simulink model "BLDC_Motor"  (R2024a)
settings: Solver=VariableStepAuto  StartTime=0.0  StopTime=10.0  RelTol=1e-3
undefined symbols (not defined in the file): Ion, Lithium
libraries: spsMosfetLib x6, spsBatteryLib x1, slpidlib x1, spsPermanentMagnetSynchronousMachineLib x1, sps_lib x1
settings Model: SimulationMode=accelerator  Creator=RGUKT  LastModifiedBy=RGUKT

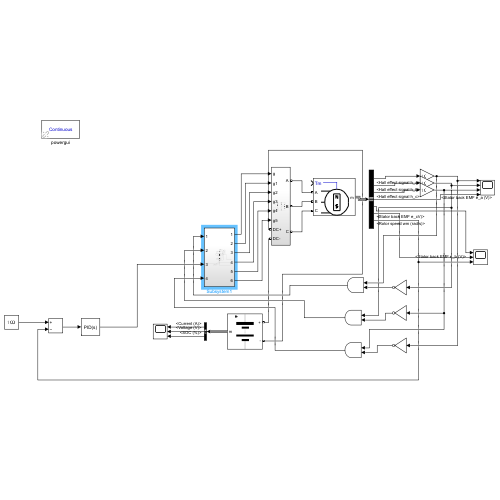
[thumbnail: Simulink's stored preview of the top-level diagram]
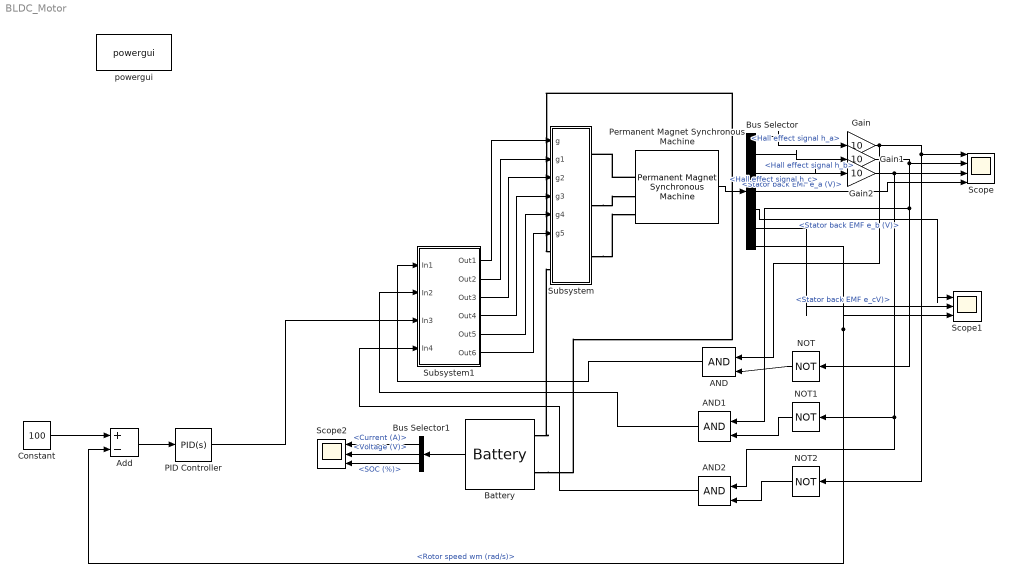
== system BLDC_Motor ==
  AND : Logic  IconShape=distinctive  AllPortsSameDT=off  OutDataTypeStr=boolean
  AND1 : Logic  IconShape=distinctive  AllPortsSameDT=off  OutDataTypeStr=boolean
  AND2 : Logic  IconShape=distinctive  AllPortsSameDT=off  OutDataTypeStr=boolean
  Add : Sum  Inputs=+-
  Battery : spsBatteryLib/Battery  BatType=Lithium-Ion  ShowTempParam=off  ThermalPreset=no  ShowAgeParam=off  NomV=7.2  NomQ=5.4  SOC=100  Batt_Tr=30  PresetModel=on  MaxQ=5.4  MinV=5.4  FullV=8.3807  Dis_rate=2.3478  R=0.013333  Normal_OP=4.8835  expZone="[7.7788      0.2653]"  current=[6.5 13 32.5]  Units=Time  Tci=20  NomT=20  T2=-30  MaxQ2=4.8  FullV2=7.1  Normal_OP2=5.655  expZone2="[6.58           1]"  Rca=0.6  ti=2000  Dp=0  Neq0=0  Tsim=1e6  Ta1=25  Qeol=5.4*0.9  Reol=0.013333*1.2  Char_age=[2.3478, 3]  Dis_age=[2.3478, 10]  N1=1500  N2=10500  N3=1000  N4=1400  Ta2=45  N5=950
  Bus Selector : BusSelector  OutputSignals=Hall effect signal h_a,Hall effect signal h_b,Hall effect signal h_c,Stator back EMF e_a (V),Stator back EMF e_b (V),Stator back EMF e_cV),Rotor speed wm (rad/s)
  Bus Selector1 : BusSelector  OutputSignals=Current (A),Voltage (V),SOC (%)
  Constant : Constant  Value=100
  Gain : Gain  Gain=10
  Gain1 : Gain  Gain=10
  Gain2 : Gain  Gain=10
  NOT : Logic  Operator=NOT  IconShape=distinctive  AllPortsSameDT=off  OutDataTypeStr=boolean
  NOT1 : Logic  Operator=NOT  IconShape=distinctive  AllPortsSameDT=off  OutDataTypeStr=boolean
  NOT2 : Logic  Operator=NOT  IconShape=distinctive  AllPortsSameDT=off  OutDataTypeStr=boolean
  PID Controller : slpidlib/PID Controller  Controller=PID  Form=Parallel  TimeDomain=Continuous-time  UseExternalTs=off  SampleTime=-1  IntegratorMethod=Forward Euler  FilterMethod=Forward Euler  ControllerParametersSource=internal  P=1  I=1  UseKiTs=off  D=0  UseExternalDerivativeSource=off  N=100  UseFilter=on  TunerSelectOption=Transfer Function Based (PID Tuner App)  InitialConditionSource=internal  InitialConditionForIntegrator=0  InitialConditionForFilter=0  DifferentiatorICPrevScaledInput=0  ExternalReset=none  TrackingMode=off  Kt=1  LimitOutput=off  SatLimitsSource=internal  UpperSaturationLimit=inf  LowerSaturationLimit=-inf  LinearizeAsGain=on  AntiWindupMode=none  Kb=1  LimitIntegrator=off  UpperIntegratorSaturationLimit=inf  LowerIntegratorSaturationLimit=-inf  POutMin=[]  POutMax=[]  IOutMin=[]  IOutMax=[]  DOutMin=[]  DOutMax=[]  NOutMin=[]  NOutMax=[]  SumOutMin=[]  SumOutMax=[]  SaturationOutMin=[]  SaturationOutMax=[]  PParamMin=[]  PParamMax=[]  IParamMin=[]  IParamMax=[]  DParamMin=[]  DParamMax=[]  NParamMin=[]  NParamMax=[]  KbParamMin=[]  KbParamMax=[]  KtParamMin=[]  KtParamMax=[]  KbOutMin=[]  KbOutMax=[]  KtOutMin=[]  KtOutMax=[]  IntegratorOutMin=[]  IntegratorOutMax=[]  FilterOutMin=[]  FilterOutMax=[]  SumI1OutMin=[]  SumI1OutMax=[]  SumI2OutMin=[]  SumI2OutMax=[]  SumI3OutMin=[]  SumI3OutMax=[]  SumI4OutMin=[]  SumI4OutMax=[]  SumDOutMin=[]  SumDOutMax=[]  DifferentiatorOutMin=[]  DifferentiatorOutMax=[]  FilterDiffOutCoefMin=[]  FilterDiffOutCoefMax=[]  ReciprocalOutMin=[]  ReciprocalOutMax=[]  SumDenOutMin=[]  SumDenOutMax=[]  SumNumOutMin=[]  SumNumOutMax=[]  DivideOutMin=[]  DivideOutMax=[]  UdiffTsProdOutMin=[]  UdiffTsProdOutMax=[]  NTsProdOutMin=[]  NTsProdOutMax=[]  UintegralTsProdOutMin=[]  UintegralTsProdOutMax=[]  UngainTsProdOutMin=[]  UngainTsProdOutMax=[]  ClampingZeroOutDataTypeStr=Inherit: Inherit via back propagation  ClampingZeroOutMin=[]  ClampingZeroOutMax=[]  FilterDenConstantOutDataTypeStr=Inherit: Inherit via back propagation  FilterDenConstantOutMin=[]  FilterDenConstantOutMax=[]  PCopyOutDataTypeStr=Inherit: Inherit via back propagation  PCopyOutMin=[]  PCopyOutMax=[]  NCopyOutDataTypeStr=Inherit: Inherit via back propagation  NCopyOutMin=[]  NCopyOutMax=[]  IntegratorContinuousStateAttributes=''  IntegratorStateMustResolveToSignalObject=off  IntegratorRTWStateStorageClass=Auto  FilterContinuousStateAttributes=''  FilterStateMustResolveToSignalObject=off  FilterRTWStateStorageClass=Auto  ParallelPVariant=InternalParameters  IdealPVariant=Disabled  IVariant=InternalParameters  DVariant=InternalParameters  IntegratorVariant=Continuous  SatVariant=Disabled  AWVariant=Passthrough  PCopyVariant=Disabled  TRVariant=Disabled  FdbkBlocksVariant=Forward  IdealPFdbkVariant=Disabled  SatFdbkVariant=Disabled  DerivativeFilterVariant=ContFilter  NVariant=InternalParameters  NCopyVariant=Disabled  FilterICVariant=InternalICsFilter  IntegratorICVariant=InternalICs  ExternalResetVariant=Disabled  TRSumVariant=Passthrough  SumFdbkVariant=Disabled  SumVariant=Sum_PID  TsampFilterVariant=InternalTs  TsampNgainVariant=Passthrough  TsampIntegralVariant=Disabled_SignalSpec  ExternalSaturationOutDataTypeStr=Inherit: Same as second input  DerivativeSourceVariant=ErrorSignal
  Permanent Magnet Synchronous Machine : spsPermanentMagnetSynchronousMachineLib/Permanent Magnet Synchronous Machine  NbPhases=3  FluxDistribution=Trapezoidal  RotorType=Round  MechanicalLoad=Torque Tm  PresetModel=No  ShowDetailedParameters=on  MeasurementBus=off  Resistance=0.0485  Inductance=8.5e-3  dqInductances=[8.5e-3,8.5e-3]  La=0.000395  MachineConstant=Flux linkage established by magnets (V.s)  Flux=0.1194  VoltageCst=100.0283  TorqueCst=0.9552  Flat=120  Mechanical=[0.0027 0.0004924 4 0]  PolePairs=4  InitialConditions=[0,0, 0,0]  InitialConditions5ph=[0 0 0 0 0 0]  RefAngle=90 degrees behind phase A axis (modified Park)  IterativeDiscreteModel=Trapezoidal non iterative  TsBlock=-1  TsPowergui=0
  Scope : Scope  NumInputPorts=4
  Scope1 : Scope  NumInputPorts=3
  Scope2 : Scope  NumInputPorts=3
  Subsystem : Subsystem
  Subsystem1 : Subsystem
  powergui : sps_lib/powergui  Priority=1  SimulationMode=Continuous  SampleTime=50e-6  frequency=60  Iterations=50  frequencyindice=0  Pbase=100e6  ErrMax=1e-4  UnitsV=kV  UnitsW=MW  buscounter=0  FunctionMessages=off  echomessages=off  EnableUseOfTLC=off  CurrentSourceSwitches=off  DisableSnubberDevices=off  DisableRonSwitches=off  DisableVfSwitches=off  DisplayEquations=off  AutomaticDiscreteSolvers=off  SolverType=Tustin/Backward Euler (TBE)  Interpol=off  ExternalGateDelay=off  methode=off  Ts=100  x0status=blocks  SPID=on  SwTol=0  HookPort=off  NonlinearTolerance=1e-4  nMaxIteration=100  ContinueOnMaxIteration=off  RestoreLinks=warning  ResistiveCurrentMeasurement=off  Frange=[0:2:500]  Ylog=off  Xlog=on  ShowGrid=off  save=off  variable=ZData  structure=0  ZoomFFT=off  StartTime=0.0  cycles=1  DisplayStyle=1  fundamental=60  FreqAxis=off  MaxFrequency=1000  frequencyindicesteady=1  RmsSteady=1  display=off
  wires:
  Permanent Magnet Synchronous Machine/1 -> Bus Selector/1
  Bus Selector/5 -> Scope1/1  "<Stator back EMF e_b (V)>"
  Bus Selector/6 -> Scope1/2  "<Stator back EMF e_cV)>"
  Bus Selector/7 -> Add/2, Scope1/3  "<Rotor speed wm (rad/s)>"
  Bus Selector/4 -> Scope/4  "<Stator back EMF e_a (V)>"
  Bus Selector/1 -> Gain/1  "<Hall effect signal h_a>"
  Bus Selector/2 -> Gain1/1  "<Hall effect signal h_b>"
  Bus Selector/3 -> Gain2/1  "<Hall effect signal h_c>"
  Gain/1 -> AND/1, NOT2/1, Scope/1
  Gain1/1 -> AND1/1, NOT/1, Scope/2
  Gain2/1 -> NOT1/1, AND2/1, Scope/3
  NOT/1 -> AND/2
  NOT2/1 -> AND2/2
  NOT1/1 -> AND1/2
  Constant/1 -> Add/1
  Add/1 -> PID Controller/1
  AND/1 -> Subsystem1/1(In1)
  AND1/1 -> Subsystem1/2(In2)
  PID Controller/1 -> Subsystem1/3(In3)
  AND2/1 -> Subsystem1/4(In4)
  Subsystem1/1(Out1) -> Subsystem/1(g)
  Subsystem1/2(Out2) -> Subsystem/2(g1)
  Subsystem1/3(Out3) -> Subsystem/3(g2)
  Subsystem1/4(Out4) -> Subsystem/4(g3)
  Subsystem1/5(Out5) -> Subsystem/5(g4)
  Subsystem1/6(Out6) -> Subsystem/6(g5)
  Battery/1 -> Bus Selector1/1
  Bus Selector1/1 -> Scope2/1  "<Current (A)>"
  Bus Selector1/2 -> Scope2/2  "<Voltage (V)>"
  Bus Selector1/3 -> Scope2/3  "<SOC (%)>"
  connections:
  Battery/LConn2 -- Subsystem/LConn1
  Battery/LConn1 -- Subsystem/LConn2
  Permanent Magnet Synchronous Machine/LConn1 -- Subsystem/RConn1
  Subsystem/RConn2 -- Permanent Magnet Synchronous Machine/LConn2
  Subsystem/RConn3 -- Permanent Magnet Synchronous Machine/LConn3

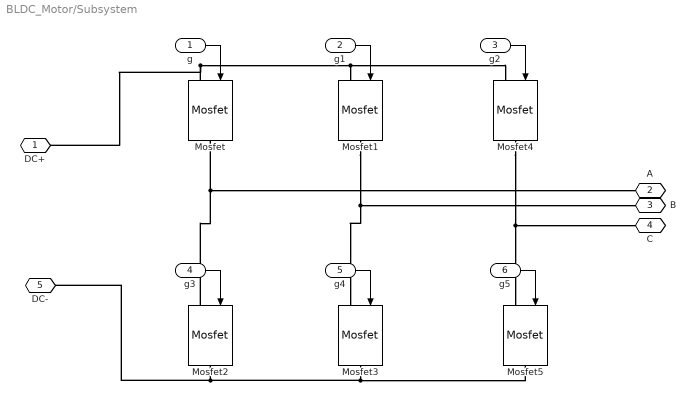
== system BLDC_Motor/Subsystem ==
  g : Inport
  g1 : Inport  Port=2
  g2 : Inport  Port=3
  g3 : Inport  Port=4
  g4 : Inport  Port=5
  g5 : Inport  Port=6
  Mosfet{,1..5} (6 alike) : spsMosfetLib/Mosfet  Ron=0.1  Lon=0  Rd=0.01  Vfd=0  IC=0  Rs=1e5  Cs=inf  Measurements=off
  DC+ : PMIOPort  Side=Left
  A : PMIOPort  Port=2  Side=Right
  B : PMIOPort  Port=3  Side=Right
  C : PMIOPort  Port=4  Side=Right
  DC- : PMIOPort  Port=5  Side=Left
  wires:
  g2/1 -> Mosfet4/1
  g4/1 -> Mosfet3/1
  g/1 -> Mosfet/1
  g1/1 -> Mosfet1/1
  g5/1 -> Mosfet5/1
  g3/1 -> Mosfet2/1
  connections:
  Mosfet2/LConn1 -- Mosfet/RConn1 -- A/RConn1
  Mosfet1/RConn1 -- B/RConn1 -- Mosfet3/LConn1
  Mosfet3/RConn1 -- DC-/RConn1 -- Mosfet2/RConn1 -- Mosfet5/RConn1
  Mosfet4/RConn1 -- Mosfet5/LConn1 -- C/RConn1
  Mosfet/LConn1 -- DC+/RConn1 -- Mosfet4/LConn1 -- Mosfet1/LConn1

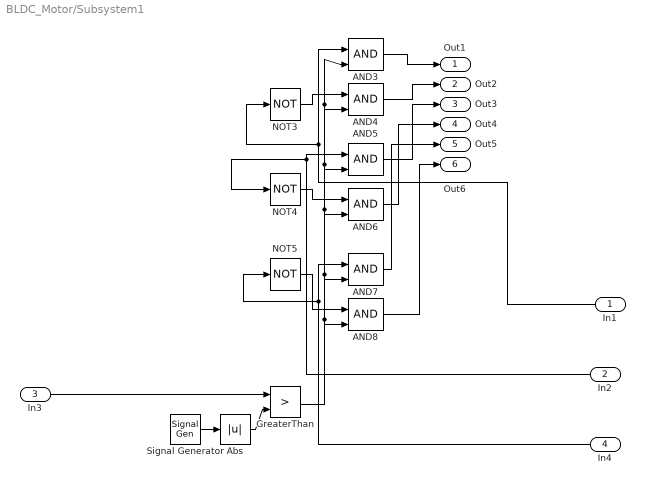
== system BLDC_Motor/Subsystem1 ==
  In1 : Inport
  In2 : Inport  Port=2
  In3 : Inport  Port=3
  In4 : Inport  Port=4
  AND{3..8} (6 alike) : Logic  IconShape=distinctive  AllPortsSameDT=off  OutDataTypeStr=boolean
  Abs : Abs  SaturateOnIntegerOverflow=off
  GreaterThan : RelationalOperator  Operator=>  OutDataTypeStr=boolean  RndMeth=Simplest  InputSameDT=off
  NOT3 : Logic  Operator=NOT  IconShape=distinctive  AllPortsSameDT=off  OutDataTypeStr=boolean
  NOT4 : Logic  Operator=NOT  IconShape=distinctive  AllPortsSameDT=off  OutDataTypeStr=boolean
  NOT5 : Logic  Operator=NOT  IconShape=distinctive  AllPortsSameDT=off  OutDataTypeStr=boolean
  Signal Generator : SignalGenerator  Units=rad/sec
  Out1 : Outport
  Out2 : Outport  Port=2
  Out3 : Outport  Port=3
  Out4 : Outport  Port=4
  Out5 : Outport  Port=5
  Out6 : Outport  Port=6
  wires:
  In3/1 -> GreaterThan/1
  In1/1 -> AND3/1, NOT3/1
  GreaterThan/1 -> AND8/2, AND7/2, AND6/2, AND5/2, AND4/2, AND3/2
  In4/1 -> AND7/1, NOT5/1
  NOT5/1 -> AND8/1
  NOT4/1 -> AND6/1
  In2/1 -> NOT4/1, AND5/1
  NOT3/1 -> AND4/1
  Abs/1 -> GreaterThan/2
  AND5/1 -> Out3/1
  AND6/1 -> Out4/1
  Signal Generator/1 -> Abs/1
  AND8/1 -> Out6/1
  AND3/1 -> Out1/1
  AND4/1 -> Out2/1
  AND7/1 -> Out5/1
